simulink model "eVTOL_System"  (R2024b)
settings: Solver=FixedStepAuto  StartTime=0.0  StopTime=inf  RelTol=1e-3
undefined symbols (not defined in the file): airspeed, Battery, BCE12, BCE_Set_init, BMS_Controller_State, C, Cell10_P, Cell11_P, Cell12_P, Cell13_P, Cell14_P, Cell15_P, Cell16_P, Cell17_P, Cell18_P, Cell19_P, Cell1_N, Cell1_P, Cell20_P, Cell21_P, Cell22_P, Cell23_P, Cell24_P, Cell2_P, Cell3_P, Cell4_P, Cell5_P, Cell6_P, Cell7_P, Cell8_P, Cell9_P, Charging_State, CityMission, control, controlParams, ControlSampleTime, CriticalTiltAngle, currentFactor, CV_Gain, ddx, ddy, ddz, Device_01, Device_02, DiscIntNeverNeededParam, dx, dy, dz, Earth, env, F, F28379D_ADC_MaxCount, F28379D_ADC_Vmax, FixedWingMission, flightState, Foc_Ki_IxTcpu, Foc_Ki_S, Foc_Kp_I, Foc_Kp_S, fractalcoef ... (+68)
libraries: fl_lib x1115, nesl_utility x617, slrealtimeethercatlib x217, simulink x130, canmsglib x101, speedgoatlib_IO611_obsolete x91, slpidlib x49, mcbcontrolslib x44, slrealtimeutilitieslib x35, speedgoatlib_hdlCoder_IO3xx x31, dspstat3 x24, mcbpositiondecoderlib x12
(part 1 of 31)
settings Model: DataDictionary=VTOLDynamicsData.sldd  Creator=The MathWorks, Inc.  LastModifiedBy=jatin.anand
settings SolverCC: ConcurrentTasks=on  PositivePriorityOrder=on  AutoInsertRateTranBlk=on
settings OptimizationCC: BlockReduction=off  OptimizeBlockIOStorage=off  EnhancedBackFolding=on  PassReuseOutputArgsThreshold=0  OptimizeBlockOrder=speed  DifferentSizesBufferReuse=on
settings DebuggingCC: TasksWithSamePriorityMsg=none  ParameterTunabilityLossMsg=error
settings HardwareCC: ProdBitPerLong=64  ProdLongLongMode=on  ProdHWDeviceType=Intel->x86-64 (Linux 64)
settings RTWCC: Description=Speedgoat Real-Time Target Machine  SystemTargetFile=speedgoat.tlc  TemplateMakefile=slrealtime_default_tmf  Toolchain=Simulink Real-Time Toolchain  BuildConfiguration=Faster Runs  CodeExecutionProfiling=on  TargetLang=C++  GPUComputeCapability=3.5
settings CodeAppCC: ForceParamTrailComments=on  OperatorAnnotations=on
settings SimulinkRealTimeTargetCC: InstructionSetFMA=off  LogToMDFFile=off

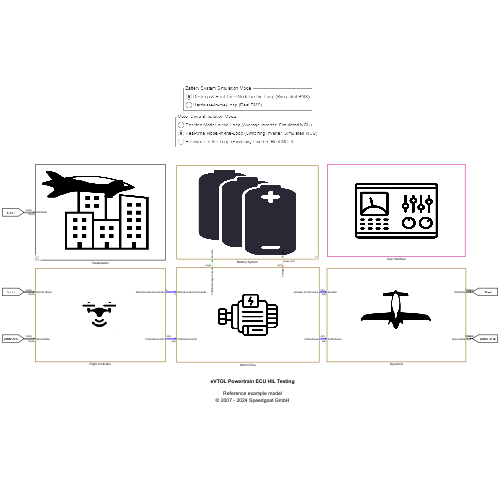
[thumbnail: Simulink's stored preview of the top-level diagram]
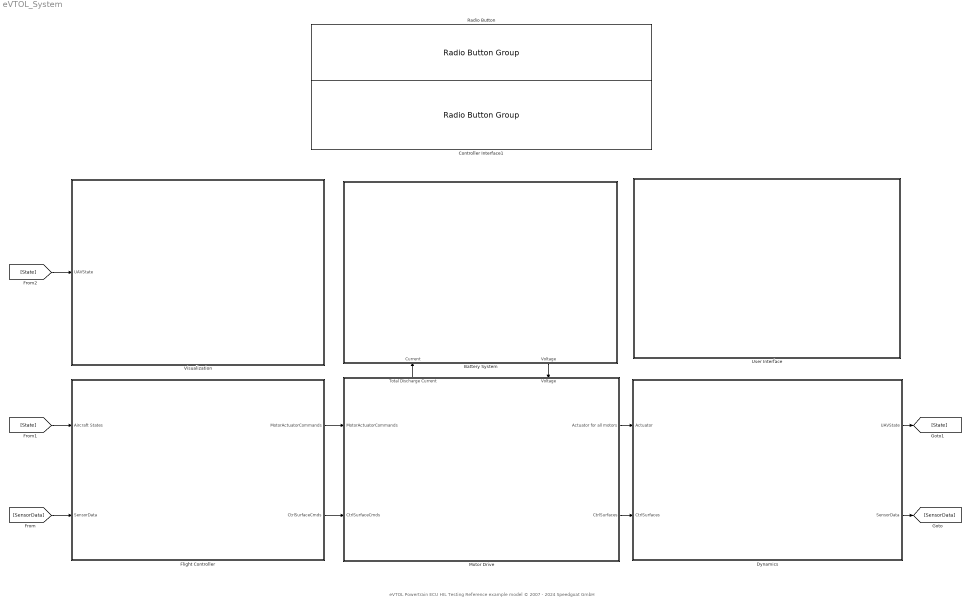
== system eVTOL_System ==
  note: eVTOL Powertrain ECU HIL Testing
      |
      | Reference example model
      | © 2007 - 2024 Speedgoat GmbH
  Battery System : Subsystem
      settings: PortSchema="{\"entries\":[{\"content\":{\"sides\":[{\"content\":{},\"type\":\"ConnectorPlacement.EquallySpacedRectSide\",\"uuid\":\"31833601-2311-4886-a109-2c0986e73e51\"},{\"content\":{\"side\":\"RIGHT\"},\"type\":\"ConnectorPlacement.EquallySpacedRectSide\",\"uuid\":\"85d08f94-66a0-4dc1-8c2a-87d8bd35677a\"},{\"content\":{\"side\":\"TOP\"},\"type\":\"ConnectorPlacement.EquallySpacedRectSide\",\"uuid\":\"8127f2a5-c494-4abc-920f-c6b2b4ea5251\"},{\"content\":{\"connectorIds\":[\"In1\",\"Out1\"],\"side\":\"BOTTOM\"},\"type\":\"ConnectorPlacement.EquallySpacedRectSide\",\"uuid\":\"983fb099-1c21-4d2b-9dd6-d2e6655b3784\"}]},\"type\":\"ConnectorPlacement.EquallySpacedConnector\",\"uuid\":\"c8b985e5-7cab-42e7-873f-ff2e7ab90a73\"}],\"packageUris\":[\"http://schema.mathworks.com/mf0/Connector/R2020b\"],\"version\":\"1.0\"}"
      mask Display: image('Battery.png');
  Controller Interface1 : RadioButtonGroup  LabelPosition=Hide  SelectedLabel=Real-time Model-in-the-Loop (Switching Inverter, Simulated MCU)  ButtonGroupName=Motor Drive Simulation Mode
      settings: Values={{'Desktop Model-in-the-Loop (Average Inverter, Simulated MCU)', 'Real-time Model-in-the-Loop (Switching Inverter, Simulated MCU)', 'Hardware-in-the-Loop (Switching Inverter, Real MCU)'}, [1 2 3]}
  Dynamics : Subsystem
      mask Display: image('fLIGHT_dYNAMICS.png', [0,0,0,0,80,80]);
  Flight Controller : Subsystem
      mask Display: image('Flight.png', [0,0,0,0,40,40]);
  Motor Drive : Subsystem
      settings: PortSchema="{\"entries\":[{\"content\":{\"sides\":[{\"content\":{\"connectorIds\":[\"In1\",\"In2\"]},\"type\":\"ConnectorPlacement.EquallySpacedRectSide\",\"uuid\":\"8efb4856-e5e8-4119-b327-f21a1b3c8e4f\"},{\"content\":{\"connectorIds\":[\"Out1\",\"Out2\"],\"side\":\"RIGHT\"},\"type\":\"ConnectorPlacement.EquallySpacedRectSide\",\"uuid\":\"1db0dfc6-79ae-47c2-8aa8-e6c666fa7b0e\"},{\"content\":{\"connectorIds\":[\"Out3\",\"In3\"],\"side\":\"TOP\"},\"type\":\"ConnectorPlacement.EquallySpacedRectSide\",\"uuid\":\"2682ef6f-b09c-4157-ad22-73f596ffc247\"}]},\"type\":\"ConnectorPlacement.EquallySpacedConnector\",\"uuid\":\"885b870f-d4fa-4030-b106-4e1ba5f331f5\"}],\"packageUris\":[\"http://schema.mathworks.com/mf0/Connector/R2020b\"],\"version\":\"1.0\"}"
      mask Display: image('PmsmMask.png');
  Radio Button : RadioButtonGroup  LabelPosition=Hide  SelectedLabel=Desktop & Real-Time Model-in-the-Loop (Simulated BMS)  ButtonGroupName=Battery System Simulation Mode
      settings: Values={{'Desktop & Real-Time Model-in-the-Loop (Simulated BMS)', 'Hardware-in-the-Loop (Real BMS)'}, [0 1]}
  User Interface : Subsystem
      mask Display: image('UIMask.png');
  Visualization : Subsystem  Variant=on  VariantControl=Visualization
      mask Display: image('3DVisualization.png');
  wires:
  Dynamics/2(SensorData) -> [SensorData]
  [SensorData] -> Flight Controller/2(SensorData)
  [State] -> Flight Controller/1(Aircraft States)
  [State] -> Visualization/1(UAVState)
  Flight Controller/1(MotorActuatorCommands) -> Motor Drive/1(MotorActuatorCommands)
  Flight Controller/2(CtrlSurfaceCmds) -> Motor Drive/2(CtrlSurfaceCmds)
  Motor Drive/1(Actuator for all motors) -> Dynamics/1(Actuator)
  Motor Drive/2(CtrlSurfaces) -> Dynamics/2(CtrlSurfaces)
  Battery System/1(Voltage) -> Motor Drive/3(Voltage)
  Dynamics/1(UAVState) -> [State]
  Motor Drive/3(Total Discharge Current) -> Battery System/1(Current)

== system eVTOL_System/Battery System ==
  note: Battery Management System HIL
      |
      | Reference example model
      | © 2007 - 2024 Speedgoat GmbH
  Current : Inport
  BMS : Subsystem  Variant=on  VariantControl=Choice
      mask Display: image('BMS.png'); % Use "Edit Image" on toolstrip to change.
  Battery : Subsystem
      mask Display: image('battery.png'); % Use "Edit Image" on toolstrip to change.
  Instrumentation : Subsystem
      mask Display: image('tunable.png'); % Use "Edit Image" on toolstrip to change.
  Voltage : Outport
  tag scope: Controller_Info=global, Controller_Output=global, Sensor_Values=global
  wires:
  [Voltage] -> Voltage/1
  [State_Request] -> BMS/1(State_Request)
  [Current_Request] -> Battery/1(Current_Request)
  BMS/1(Controller_Info) -> [Controller_Info]  "Controller_Info"
  Battery/1(Sensor_Values) -> [Sensor_Values]
  BMS/2(Controller_Output) -> [Controller_Output]  "Controller_Output"
  Current/1 -> Instrumentation/1(Current)
  [Sensor_Values] -> BMS/2(Sensor_Values)
  connections:
  Battery/RConn1 -- BMS/LConn1
  Battery/RConn2 -- BMS/LConn2
  Battery/RConn3 -- BMS/LConn3

== system eVTOL_System/Dynamics ==
  note: Forces and Moments - VTOL UAV plant model and weather model
      | 6DOF (Euler Angles Conversion) - Converts forces and moments from body to inertial frame
      | Ground Truth Bus - converts UAV States into bus
  Actuator : Inport
  CtrlSurfaces : Inport  Port=2
  6DOF (Euler Angles)1 : shared6dof/6DOF (Euler Angles)  units=Metric (MKS)  mtype=Fixed  rep=Euler Angles  xme_0=[xGround, yGround, zGround]  Vm_0=[vIni 0 0]  eul_0=[iniRoll initPitch iniYaw]  pm_0=[0 0 0]  mass_0=6.031  mass_e=0.5  mass_f=2.0  inertia=[uavParam.geom.Ixx 0 0; 0 uavParam.geom.Iyy 0; 0 0 uavParam.geom.Izz]  inertia_e=eye(3)  inertia_f=2*eye(3)  k_quat=1.0  vre_flag=on  abi_flag=on  aMode=0  xme_statename=''  Vm_statename=''  eul_statename=''  quat_statename=''  pm_statename=''  mass_statename=''
  Bus Selector : BusSelector  OutputSignals=RotorParameters.w1,RotorParameters.w2,RotorParameters.w3,RotorParameters.w4
  Force and Moments : Subsystem
  Ground Truth Bus : Subsystem
  Scope : Scope  NumInputPorts=4
  Terminator : Terminator
  Variant Subsystem : Subsystem  Variant=on  VariantControl=Choice
  UAVState : Outport
  SensorData : Outport  Port=2
  wires:
  Force and Moments/1(F) -> 6DOF (Euler Angles)1/1
  Force and Moments/2(M) -> 6DOF (Euler Angles)1/2
  Actuator/1 -> Force and Moments/1(Actuator)
  CtrlSurfaces/1 -> Force and Moments/2(CtrlSurfaces)
  6DOF (Euler Angles)1/1 -> Ground Truth Bus/1(Ve)  "Ve"
  6DOF (Euler Angles)1/2 -> Ground Truth Bus/2(Xe)  "Xe"
  6DOF (Euler Angles)1/3 -> Ground Truth Bus/3(Euler)  "Euler"
  6DOF (Euler Angles)1/4 -> Ground Truth Bus/4(DCMbe)  "DCMbe"
  6DOF (Euler Angles)1/5 -> Ground Truth Bus/5(Vb)  "Vb"
  6DOF (Euler Angles)1/6 -> Ground Truth Bus/6(pqr)  "pqr"
  6DOF (Euler Angles)1/7 -> Terminator/1
  6DOF (Euler Angles)1/8 -> Ground Truth Bus/7(Abb)  "Abb"
  Force and Moments/3(RotorParams) -> Ground Truth Bus/9(RotorParams)  "RotorParams"
  Force and Moments/4(AirData) -> Ground Truth Bus/10(AirData)
  Variant Subsystem/1(SensorData) -> SensorData/1
  6DOF (Euler Angles)1/9 -> Ground Truth Bus/8(Abe)
  Ground Truth Bus/1(Ground Truth) -> Bus Selector/1, UAVState/1, Force and Moments/3(States), Variant Subsystem/1(UAVStates)  "Ground Truth"
  Bus Selector/1 -> Scope/1  "<w1>"
  Bus Selector/2 -> Scope/2  "<w2>"
  Bus Selector/3 -> Scope/3  "<w3>"
  Bus Selector/4 -> Scope/4  "<w4>"

== system eVTOL_System/Flight Controller ==
  Aircraft States : Inport
  SensorData : Inport  Port=2
  Autopilot : Subsystem
  Estimator : Subsystem  Variant=on
  Ground Control Station : Subsystem
  Guidance Test Bench : Subsystem
  MotorActuatorCommands : Outport
  CtrlSurfaceCmds : Outport  Port=2
  wires:
  Guidance Test Bench/3(AACSP) -> Autopilot/3(AAC)
  Estimator/1(EstimatedStates) -> Autopilot/6(EstimatedStates), Ground Control Station/1(UAVState)
  Ground Control Station/1(Global Mission) -> Guidance Test Bench/2(Global Mission)
  Guidance Test Bench/5(FlightMode) -> Autopilot/5(FlightMode)
  Guidance Test Bench/1(HoverSP) -> Autopilot/1(HoverCommands)
  Guidance Test Bench/2(FixedWingSP) -> Autopilot/2(FixedWingSP)
  SensorData/1 -> Estimator/1(SensorData)
  Guidance Test Bench/4(ctrlMode) -> Autopilot/4(CtrlMode)
  Autopilot/1(MotorActuatorCommands) -> MotorActuatorCommands/1
  Autopilot/2(CtrlSurfaceCmds) -> CtrlSurfaceCmds/1
  Aircraft States/1 -> Guidance Test Bench/1(Aircraft States)

== system eVTOL_System/Motor Drive ==
  MotorActuatorCommands : Inport
  CtrlSurfaceCmds : Inport  Port=2
  Voltage : Inport  Port=3
  Actuator To PWM for all motors : Subsystem
  Actuator To RPM for 1 motor : Subsystem
  Actuator To RPM for 1 motor1 : Subsystem
  Actuator To RPM for 1 motor2 : Subsystem
  Actuator To RPM for 1 motor3 : Subsystem
  Add : Sum  Inputs=++++
  Closed_Loop_FOC{,1..3} (4 alike) : Constant  OutDataTypeStr=boolean  SampleTime=Ts_UI
  Controller : Subsystem  Variant=on  VariantControl=Choice
      settings: PortSchema="{\"entries\":[{\"content\":{\"sides\":[{\"content\":{\"connectorIds\":[\"In1\",\"In2\",\"In3\",\"In4\",\"In5\",\"In6\"]},\"type\":\"ConnectorPlacement.EquallySpacedRectSide\",\"uuid\":\"39f08c92-b87f-4f95-877f-fef0e466fbdb\"},{\"content\":{\"connectorIds\":[\"Out1\"],\"side\":\"RIGHT\"},\"type\":\"ConnectorPlacement.EquallySpacedRectSide\",\"uuid\":\"6fadd6f2-7db3-41c1-89a7-be1692c18c49\"},{\"content\":{\"connectorIds\":[\"Out2\"],\"side\":\"TOP\"},\"type\":\"ConnectorPlacement.EquallySpacedRectSide\",\"uuid\":\"aea4ee68-7094-4bdc-b416-2d8969306971\"}]},\"type\":\"ConnectorPlacement.EquallySpacedConnector\",\"uuid\":\"e129f01f-1291-4735-8ea4-164650c1b4f8\"}],\"packageUris\":[\"http://schema.mathworks.com/mf0/Connector/R2020b\"],\"version\":\"1.0\"}"
      mask Display: image('MCUMask.png');
  Controller Parameters : Subsystem
  Controller Parameters1 : Subsystem
  Controller Parameters2 : Subsystem
  Controller Parameters3 : Subsystem
  Controller1 : Subsystem  Variant=on  VariantControl=Choice
      settings: PortSchema="{\"entries\":[{\"content\":{\"sides\":[{\"content\":{\"connectorIds\":[\"In1\",\"In2\",\"In3\",\"In4\",\"In5\",\"In6\"]},\"type\":\"ConnectorPlacement.EquallySpacedRectSide\",\"uuid\":\"39f08c92-b87f-4f95-877f-fef0e466fbdb\"},{\"content\":{\"connectorIds\":[\"Out1\"],\"side\":\"RIGHT\"},\"type\":\"ConnectorPlacement.EquallySpacedRectSide\",\"uuid\":\"6fadd6f2-7db3-41c1-89a7-be1692c18c49\"},{\"content\":{\"connectorIds\":[\"Out2\"],\"side\":\"TOP\"},\"type\":\"ConnectorPlacement.EquallySpacedRectSide\",\"uuid\":\"aea4ee68-7094-4bdc-b416-2d8969306971\"}]},\"type\":\"ConnectorPlacement.EquallySpacedConnector\",\"uuid\":\"e129f01f-1291-4735-8ea4-164650c1b4f8\"}],\"packageUris\":[\"http://schema.mathworks.com/mf0/Connector/R2020b\"],\"version\":\"1.0\"}"
      mask Display: image('MCUMask.png');
  Controller2 : Subsystem  Variant=on  VariantControl=Choice
      settings: PortSchema="{\"entries\":[{\"content\":{\"sides\":[{\"content\":{\"connectorIds\":[\"In1\",\"In2\",\"In3\",\"In4\",\"In5\",\"In6\"]},\"type\":\"ConnectorPlacement.EquallySpacedRectSide\",\"uuid\":\"39f08c92-b87f-4f95-877f-fef0e466fbdb\"},{\"content\":{\"connectorIds\":[\"Out1\"],\"side\":\"RIGHT\"},\"type\":\"ConnectorPlacement.EquallySpacedRectSide\",\"uuid\":\"6fadd6f2-7db3-41c1-89a7-be1692c18c49\"},{\"content\":{\"connectorIds\":[\"Out2\"],\"side\":\"TOP\"},\"type\":\"ConnectorPlacement.EquallySpacedRectSide\",\"uuid\":\"aea4ee68-7094-4bdc-b416-2d8969306971\"}]},\"type\":\"ConnectorPlacement.EquallySpacedConnector\",\"uuid\":\"e129f01f-1291-4735-8ea4-164650c1b4f8\"}],\"packageUris\":[\"http://schema.mathworks.com/mf0/Connector/R2020b\"],\"version\":\"1.0\"}"
      mask Display: image('MCUMask.png');
  Controller3 : Subsystem  Variant=on  VariantControl=Choice
      settings: PortSchema="{\"entries\":[{\"content\":{\"sides\":[{\"content\":{\"connectorIds\":[\"In1\",\"In2\",\"In3\",\"In4\",\"In5\",\"In6\"]},\"type\":\"ConnectorPlacement.EquallySpacedRectSide\",\"uuid\":\"39f08c92-b87f-4f95-877f-fef0e466fbdb\"},{\"content\":{\"connectorIds\":[\"Out1\"],\"side\":\"RIGHT\"},\"type\":\"ConnectorPlacement.EquallySpacedRectSide\",\"uuid\":\"6fadd6f2-7db3-41c1-89a7-be1692c18c49\"},{\"content\":{\"connectorIds\":[\"Out2\"],\"side\":\"TOP\"},\"type\":\"ConnectorPlacement.EquallySpacedRectSide\",\"uuid\":\"aea4ee68-7094-4bdc-b416-2d8969306971\"}]},\"type\":\"ConnectorPlacement.EquallySpacedConnector\",\"uuid\":\"e129f01f-1291-4735-8ea4-164650c1b4f8\"}],\"packageUris\":[\"http://schema.mathworks.com/mf0/Connector/R2020b\"],\"version\":\"1.0\"}"
      mask Display: image('MCUMask.png');
  Controller_fbk_signals : Subsystem
  Controller_fbk_signals1 : Subsystem
  Controller_fbk_signals2 : Subsystem
  Controller_fbk_signals3 : Subsystem
  Data Type Conversion{,1..3} (4 alike) : DataTypeConversion  OutDataTypeStr=single  SaturateOnIntegerOverflow=off  RndMeth=Floor
  Delay{,1..3} (4 alike) : Delay
  EnablePWM{,1..3} (4 alike) : Constant  OutDataTypeStr=boolean  SampleTime=Ts_UI
  Fault Trigering : Subsystem
  Fault Trigering1 : Subsystem
  Fault Trigering2 : Subsystem
  Fault Trigering3 : Subsystem
  Load{,1..3} (4 alike) : Constant  Value=0  OutDataTypeStr=single
  Motor Model Feedback : Subsystem
  Motor Model Feedback1 : Subsystem
  Motor Model Feedback2 : Subsystem
  Motor Model Feedback3 : Subsystem
  Mux{,1..3} (4 alike) : Mux  Inputs=2
  SimulationVariant : Constant  Value=2
  Terminator{,1..4} (5 alike) : Terminator
  Three-Phase PMSM Drive : Subsystem  Variant=on  VariantControl=Choice
      settings: PortSchema="{\"entries\":[{\"content\":{\"sides\":[{\"content\":{\"connectorIds\":[\"In1\",\"In2\",\"In3\"]},\"type\":\"ConnectorPlacement.EquallySpacedRectSide\",\"uuid\":\"be3bef0c-fa0d-49a9-8d81-4a9438f9f09e\"},{\"content\":{\"connectorIds\":[\"Out1\",\"Out2\",\"Out3\",\"Out4\",\"Out5\",\"Out6\"],\"side\":\"RIGHT\"},\"type\":\"ConnectorPlacement.EquallySpacedRectSide\",\"uuid\":\"a97c4291-bd47-47ae-a87a-e148291abc4a\"},{\"content\":{\"connectorIds\":[\"In4\"],\"side\":\"TOP\"},\"type\":\"ConnectorPlacement.EquallySpacedRectSide\",\"uuid\":\"93bcf0c4-5b44-4ac3-b6c3-6b4577237bd1\"}]},\"type\":\"ConnectorPlacement.EquallySpacedConnector\",\"uuid\":\"9c4ab161-5f4a-4191-8213-47b9045836c1\"}],\"packageUris\":[\"http://schema.mathworks.com/mf0/Connector/R2020b\"],\"version\":\"1.0\"}"
      mask Display: image('pmsmMask.png'); % Use "Edit Image" on toolstrip to change.
  Three-Phase PMSM Drive1 : Subsystem  Variant=on  VariantControl=Choice
      settings: PortSchema="{\"entries\":[{\"content\":{\"sides\":[{\"content\":{\"connectorIds\":[\"In1\",\"In2\",\"In3\"]},\"type\":\"ConnectorPlacement.EquallySpacedRectSide\",\"uuid\":\"be3bef0c-fa0d-49a9-8d81-4a9438f9f09e\"},{\"content\":{\"connectorIds\":[\"Out1\",\"Out2\",\"Out3\",\"Out4\",\"Out5\",\"Out6\"],\"side\":\"RIGHT\"},\"type\":\"ConnectorPlacement.EquallySpacedRectSide\",\"uuid\":\"a97c4291-bd47-47ae-a87a-e148291abc4a\"},{\"content\":{\"connectorIds\":[\"In4\"],\"side\":\"TOP\"},\"type\":\"ConnectorPlacement.EquallySpacedRectSide\",\"uuid\":\"93bcf0c4-5b44-4ac3-b6c3-6b4577237bd1\"}]},\"type\":\"ConnectorPlacement.EquallySpacedConnector\",\"uuid\":\"9c4ab161-5f4a-4191-8213-47b9045836c1\"}],\"packageUris\":[\"http://schema.mathworks.com/mf0/Connector/R2020b\"],\"version\":\"1.0\"}"
      mask Display: image('pmsmMask.png'); % Use "Edit Image" on toolstrip to change.
  Three-Phase PMSM Drive2 : Subsystem  Variant=on  VariantControl=Choice
      settings: PortSchema="{\"entries\":[{\"content\":{\"sides\":[{\"content\":{\"connectorIds\":[\"In1\",\"In2\",\"In3\"]},\"type\":\"ConnectorPlacement.EquallySpacedRectSide\",\"uuid\":\"be3bef0c-fa0d-49a9-8d81-4a9438f9f09e\"},{\"content\":{\"connectorIds\":[\"Out1\",\"Out2\",\"Out3\",\"Out4\",\"Out5\",\"Out6\"],\"side\":\"RIGHT\"},\"type\":\"ConnectorPlacement.EquallySpacedRectSide\",\"uuid\":\"a97c4291-bd47-47ae-a87a-e148291abc4a\"},{\"content\":{\"connectorIds\":[\"In4\"],\"side\":\"TOP\"},\"type\":\"ConnectorPlacement.EquallySpacedRectSide\",\"uuid\":\"93bcf0c4-5b44-4ac3-b6c3-6b4577237bd1\"}]},\"type\":\"ConnectorPlacement.EquallySpacedConnector\",\"uuid\":\"9c4ab161-5f4a-4191-8213-47b9045836c1\"}],\"packageUris\":[\"http://schema.mathworks.com/mf0/Connector/R2020b\"],\"version\":\"1.0\"}"
      mask Display: image('pmsmMask.png'); % Use "Edit Image" on toolstrip to change.
  Three-Phase PMSM Drive3 : Subsystem  Variant=on  VariantControl=Choice
      settings: PortSchema="{\"entries\":[{\"content\":{\"sides\":[{\"content\":{\"connectorIds\":[\"In1\",\"In2\",\"In3\"]},\"type\":\"ConnectorPlacement.EquallySpacedRectSide\",\"uuid\":\"be3bef0c-fa0d-49a9-8d81-4a9438f9f09e\"},{\"content\":{\"connectorIds\":[\"Out1\",\"Out2\",\"Out3\",\"Out4\",\"Out5\",\"Out6\"],\"side\":\"RIGHT\"},\"type\":\"ConnectorPlacement.EquallySpacedRectSide\",\"uuid\":\"a97c4291-bd47-47ae-a87a-e148291abc4a\"},{\"content\":{\"connectorIds\":[\"In4\"],\"side\":\"TOP\"},\"type\":\"ConnectorPlacement.EquallySpacedRectSide\",\"uuid\":\"93bcf0c4-5b44-4ac3-b6c3-6b4577237bd1\"}]},\"type\":\"ConnectorPlacement.EquallySpacedConnector\",\"uuid\":\"9c4ab161-5f4a-4191-8213-47b9045836c1\"}],\"packageUris\":[\"http://schema.mathworks.com/mf0/Connector/R2020b\"],\"version\":\"1.0\"}"
      mask Display: image('pmsmMask.png'); % Use "Edit Image" on toolstrip to change.
  Actuator for all motors : Outport
  CtrlSurfaces : Outport  Port=2
  Total Discharge Current : Outport  Port=3
  wires:
  CtrlSurfaceCmds/1 -> CtrlSurfaces/1
  SimulationVariant/1 -> Terminator2/1
  Controller/1(Controller_fbk) -> Controller_fbk_signals/1(Controller_fbk)
  [Iab1] -> Controller/1(Iab)
  Three-Phase PMSM Drive/4(Motor_Spd) -> Motor Model Feedback/4(Motor_SPD_rads)
  Three-Phase PMSM Drive/3(Ic) -> Motor Model Feedback/3(Ic)
  [QAE_Pos_C1] -> Controller/2(QAE_MIL_fbk)
  Three-Phase PMSM Drive/2(Ib) -> Mux/2, Motor Model Feedback/2(Ib)
  Controller Parameters/1(Controller Parameters) -> Controller/6(Controller_Parameters)
  Three-Phase PMSM Drive/1(Ia) -> Mux/1, Motor Model Feedback/1(Ia)
  EnablePWM/1 -> Controller/3(EnablePWM)
  Three-Phase PMSM Drive/5(Motor_Angle) -> Terminator/1
  Load/1 -> Three-Phase PMSM Drive/3(LdTrq/Spd)
  Mux/1 -> [Iab1]
  Closed_Loop_FOC/1 -> Controller/4(Closed_Loop_FOC)
  Fault Trigering/1(Faults) -> Three-Phase PMSM Drive/2(Fault)
  Three-Phase PMSM Drive/6(QAE_Pos_C) -> [QAE_Pos_C1]
  Controller/2(Simu_config) -> Three-Phase PMSM Drive/4(Simu_config)
  Actuator To PWM for all motors/1(To PWM) -> Actuator for all motors/1
  Data Type Conversion/1 -> Controller/5(Speed_CMD_RPM)
  Three-Phase PMSM Drive1/5(Motor_Angle) -> Terminator1/1
  Load1/1 -> Three-Phase PMSM Drive1/3(LdTrq/Spd)
  Three-Phase PMSM Drive1/4(Motor_Spd) -> Motor Model Feedback1/4(Motor_SPD_rads)
  [Iab2] -> Controller1/1(Iab)
  Three-Phase PMSM Drive1/3(Ic) -> Motor Model Feedback1/3(Ic)
  Mux1/1 -> [Iab2]
  Three-Phase PMSM Drive1/2(Ib) -> Mux1/2, Motor Model Feedback1/2(Ib)
  Data Type Conversion1/1 -> Controller1/5(Speed_CMD_RPM)
  Controller Parameters1/1(Controller Parameters) -> Controller1/6(Controller_Parameters)
  Three-Phase PMSM Drive1/6(QAE_Pos_C) -> [QAE_Pos_C2]
  [QAE_Pos_C2] -> Controller1/2(QAE_MIL_fbk)
  Controller1/2(Simu_config) -> Three-Phase PMSM Drive1/4(Simu_config)
  Fault Trigering1/1(Faults) -> Three-Phase PMSM Drive1/2(Fault)
  EnablePWM1/1 -> Controller1/3(EnablePWM)
  Closed_Loop_FOC1/1 -> Controller1/4(Closed_Loop_FOC)
  Controller1/1(Controller_fbk) -> Controller_fbk_signals1/1(Controller_fbk)
  Three-Phase PMSM Drive1/1(Ia) -> Mux1/1, Motor Model Feedback1/1(Ia)
  Actuator To RPM for 1 motor1/1(RPM) -> Data Type Conversion1/1
  Controller2/1(Controller_fbk) -> Controller_fbk_signals2/1(Controller_fbk)
  Closed_Loop_FOC2/1 -> Controller2/4(Closed_Loop_FOC)
  Fault Trigering2/1(Faults) -> Three-Phase PMSM Drive2/2(Fault)
  Three-Phase PMSM Drive2/6(QAE_Pos_C) -> [QAE_Pos_C3]
  Actuator To RPM for 1 motor2/1(RPM) -> Data Type Conversion2/1
  Controller Parameters2/1(Controller Parameters) -> Controller2/6(Controller_Parameters)
  Data Type Conversion2/1 -> Controller2/5(Speed_CMD_RPM)
  Three-Phase PMSM Drive2/1(Ia) -> Mux2/1, Motor Model Feedback2/1(Ia)
  Controller2/2(Simu_config) -> Three-Phase PMSM Drive2/4(Simu_config)
  [QAE_Pos_C3] -> Controller2/2(QAE_MIL_fbk)
  Three-Phase PMSM Drive2/2(Ib) -> Mux2/2, Motor Model Feedback2/2(Ib)
  [Iab3] -> Controller2/1(Iab)
  Three-Phase PMSM Drive2/3(Ic) -> Motor Model Feedback2/3(Ic)
  Load2/1 -> Three-Phase PMSM Drive2/3(LdTrq/Spd)
  Three-Phase PMSM Drive2/4(Motor_Spd) -> Motor Model Feedback2/4(Motor_SPD_rads)
  Mux2/1 -> [Iab3]
  EnablePWM2/1 -> Controller2/3(EnablePWM)
  Three-Phase PMSM Drive2/5(Motor_Angle) -> Terminator3/1
  Controller3/1(Controller_fbk) -> Controller_fbk_signals3/1(Controller_fbk)
  Closed_Loop_FOC3/1 -> Controller3/4(Closed_Loop_FOC)
  Fault Trigering3/1(Faults) -> Three-Phase PMSM Drive3/2(Fault)
  Three-Phase PMSM Drive3/6(QAE_Pos_C) -> [QAE_Pos_C4]
  Actuator To RPM for 1 motor3/1(RPM) -> Data Type Conversion3/1
  Controller Parameters3/1(Controller Parameters) -> Controller3/6(Controller_Parameters)
  Data Type Conversion3/1 -> Controller3/5(Speed_CMD_RPM)
  Three-Phase PMSM Drive3/1(Ia) -> Mux3/1, Motor Model Feedback3/1(Ia)
  Controller3/2(Simu_config) -> Three-Phase PMSM Drive3/4(Simu_config)
  [QAE_Pos_C4] -> Controller3/2(QAE_MIL_fbk)
  Three-Phase PMSM Drive3/2(Ib) -> Mux3/2, Motor Model Feedback3/2(Ib)
  [Iab4] -> Controller3/1(Iab)
  Three-Phase PMSM Drive3/3(Ic) -> Motor Model Feedback3/3(Ic)
  Load3/1 -> Three-Phase PMSM Drive3/3(LdTrq/Spd)
  Three-Phase PMSM Drive3/4(Motor_Spd) -> Motor Model Feedback3/4(Motor_SPD_rads)
  Mux3/1 -> [Iab4]
  EnablePWM3/1 -> Controller3/3(EnablePWM)
  Three-Phase PMSM Drive3/5(Motor_Angle) -> Terminator4/1
  MotorActuatorCommands/1 -> Actuator To RPM for 1 motor1/1(Motor Commands), Actuator To RPM for 1 motor2/1(Motor Commands), Actuator To RPM for 1 motor3/1(Motor Commands), Actuator To PWM for all motors/1(Motor Commands), Actuator To RPM for 1 motor/1(Motor Commands)
  [Idc4] -> Delay3/1
  [Idc3] -> Delay2/1
  [Idc2] -> Delay1/1
  [Idc1] -> Delay/1
  Add/1 -> Total Discharge Current/1
  Delay/1 -> Add/1
  Delay1/1 -> Add/2
  Delay2/1 -> Add/3
  Delay3/1 -> Add/4
  Actuator To RPM for 1 motor/1(RPM) -> Data Type Conversion/1
  Voltage/1 -> Three-Phase PMSM Drive3/1(V_dc), Three-Phase PMSM Drive2/1(V_dc), Three-Phase PMSM Drive1/1(V_dc), Three-Phase PMSM Drive/1(V_dc)

== system eVTOL_System/User Interface ==
  " System User Interface" : Subsystem
      mask Display: image('UIMask.png');
  BMS User Interface : Subsystem
      mask Display: image('UIMask.png');
  Motor Drive User Interface : Subsystem
      mask Display: image('UIMask.png');

== system eVTOL_System/Visualization ==
  UAVState : Inport
  No Visualization : Subsystem  VariantControl=Visualization==0
  Photorealistic : Subsystem  Variant=on  VariantControl=Visualization==2
  Visualization : Subsystem  Variant=on  VariantControl=Visualization==1

== system eVTOL_System/Battery System/BMS ==
  State_Request : Inport
  Sensor_Values : Inport  Port=2
  HIL : Subsystem  VariantControl=strcmp(get_param(['eVTOL_System/Battery System/Instrumentation/Simulation_Profile_Value'], 'Value'),'1')
  MIL : Subsystem  VariantControl=strcmp(get_param(['eVTOL_System/Battery System/Instrumentation/Simulation_Profile_Value'], 'Value'),'0')
  Cells : PMIOPort  Side=Left
  Cells1 : PMIOPort  Port=2  Side=Left
  Cells2 : PMIOPort  Port=3  Side=Left
  Controller_Info : Outport
  Controller_Output : Outport  Port=2

== system eVTOL_System/Battery System/Battery ==
  Current_Request : Inport
  Battery Pack : Subsystem
  Bus Creator1 : BusCreator  Inputs=6
  Data Type Conversion{,1..3,6..7} (6 alike) : DataTypeConversion  OutDataTypeStr=single  SaturateOnIntegerOverflow=off  RndMeth=Floor
  Electrical Interface : Subsystem
      settings: PortSchema="{\"entries\":[{\"content\":{\"sides\":[{\"content\":{\"connectorIds\":[\"LConn1\",\"LConn2\"]},\"type\":\"ConnectorPlacement.EquallySpacedRectSide\",\"uuid\":\"060ff703-e9b3-40ce-a787-2ee59c0c5ac0\"},{\"content\":{\"connectorIds\":[\"Out1\",\"Out2\"],\"side\":\"RIGHT\"},\"type\":\"ConnectorPlacement.EquallySpacedRectSide\",\"uuid\":\"8c9bb67a-bc70-410b-a295-07dda5ac66bb\"},{\"content\":{\"side\":\"TOP\"},\"type\":\"ConnectorPlacement.EquallySpacedRectSide\",\"uuid\":\"38660739-cfc2-45c9-bc16-eb56669afec1\"},{\"content\":{\"connectorIds\":[\"In1\"],\"side\":\"BOTTOM\"},\"type\":\"ConnectorPlacement.EquallySpacedRectSide\",\"uuid\":\"71db0731-26a1-4041-8f3c-8f442f4d5aa6\"}]},\"type\":\"ConnectorPlacement.EquallySpacedConnector\",\"uuid\":\"4bfbaf33-58df-40e3-8b4c-5be4570a9e05\"}],\"packageUris\":[\"http://schema.mathworks.com/mf0/Connector/R2020b\"],\"version\":\"1.0\"}"
  HW Interface : Subsystem  Variant=on  VariantControl=Choice
  Override : Subsystem
  Rate Transition1 : RateTransition  OutPortSampleTime=ts_system
  Cells : PMIOPort  Side=Right
  Cells1 : PMIOPort  Port=2  Side=Right
  Cells2 : PMIOPort  Port=3  Side=Right
  Sensor_Values : Outport
  tag scope: Cells_SOCs=global
  wires:
  Current_Request/1 -> Rate Transition1/1
  Electrical Interface/1(Pack_Current) -> Data Type Conversion2/1
  Electrical Interface/2(Pack_Voltage) -> Data Type Conversion1/1
  Data Type Conversion/1 -> Bus Creator1/1  "Cell_Voltages"
  Data Type Conversion1/1 -> Bus Creator1/4  "Pack_Voltage"
  Data Type Conversion2/1 -> Bus Creator1/3  "Pack_Current"
  Data Type Conversion3/1 -> Bus Creator1/2  "Cell_Temperatures"
  [Ambient_Temperature_User] -> Battery Pack/1(Ambient_Temperature)
  Battery Pack/1(Cell_Voltages) -> Data Type Conversion/1
  Battery Pack/2(Cell_Temperatures) -> Data Type Conversion3/1
  Battery Pack/3(Cell_SOCs) -> [Cells_SOCs]  "Cell_SOCs"
  HW Interface/1(Sensor_Values_Real) -> Sensor_Values/1
  Rate Transition1/1 -> Electrical Interface/1(Current_Request)
  Bus Creator1/1 -> Override/1(Input)
  [Pack_Voltage_76Cells] -> Data Type Conversion6/1
  [Pack_Voltage_24Cells] -> Data Type Conversion7/1
  Data Type Conversion6/1 -> Bus Creator1/6  "Pack_Voltage2"
  Data Type Conversion7/1 -> Bus Creator1/5  "Pack_Voltage1"
  Override/1(Output) -> HW Interface/1(Sensor_Values_Sim)
  connections:
  Battery Pack/RConn1 -- Electrical Interface/LConn1
  Battery Pack/RConn2 -- Electrical Interface/LConn2
  Battery Pack/RConn3 -- HW Interface/LConn1
  HW Interface/RConn1 -- Cells/RConn1
  Battery Pack/RConn4 -- Cells1/RConn1
  Cells2/RConn1 -- Battery Pack/RConn5

== system eVTOL_System/Battery System/Instrumentation ==
  Current : Inport
  Ambient_Temperature : Constant  Value=25  SampleTime=-1
  Celsius_to_Kelvin : Subsystem
  Constant1 : Constant
  Current Control : Subsystem
  Instrumented Signals : Subsystem
  Mux : Mux  Inputs=3
  Simulation_Profile_Value : Constant  Value=0
  State_Request : simulink/Sources/Enumerated Constant  OutDataTypeStr=Enum: SRE  Value=SRE(0)  SampleTime=inf
  Terminator1 : Terminator
  Terminator4 : Terminator
  Test_Mode_Selector : Constant  Value=TestMode
  tag scope: Ambient_Temperature_User=global, Current_Request=global, State_Request=global
  wires:
  Celsius_to_Kelvin/1(K) -> [Ambient_Temperature_User]
  Ambient_Temperature/1 -> Celsius_to_Kelvin/1(C)
  Constant1/1 -> Current Control/2(Current_Request_User_Bypass)
  Current Control/1(Current_Request) -> [Current_Request]  "Pack_Current_Request"
  State_Request/1 -> [State_Request]
  [Controller_Output] -> Instrumented Signals/1(Controller_Output), Current Control/4(Controller_Output)
  [Controller_Info] -> Instrumented Signals/2(Controller_Info), Current Control/3(Controller_Info)
  [Sensor_Values] -> Instrumented Signals/3(Sensor_Values)
  [Cells_SOCs] -> Instrumented Signals/5(Cells_SOCs)
  Simulation_Profile_Value/1 -> Terminator4/1
  Test_Mode_Selector/1 -> Terminator1/1
  [Balancing_Currents1] -> Mux/2
  [Balancing_Currents] -> Mux/1
  [Balancing_Currents2] -> Mux/3
  Mux/1 -> Instrumented Signals/4(Balancing_Currents)
  Current/1 -> Current Control/1(Current_Request_User)

== system eVTOL_System/Dynamics/Force and Moments ==
  note: Weather Model - Wind model is disabled by default. To enable wind model, run Wind = 0 and configure the wind model in the Weather Model subsystem.
      |
      | Aerodynamic Forces - Computes aerodynamic forces of the UAV. To modify the aerodynamic derivatives of the UAV, modify the uavParam.aero struct with your own data, or use the Aerodynamic Forces and Moments block from Aerospace Blockset
      |
      | Propulsion - Models the propulsion system. Open this subsystem to configure the rotor direction, tilt angle, etc.
  Actuator : Inport
  CtrlSurfaces : Inport  Port=2
  States : Inport  Port=3
  Add : Sum  Inputs=++++
  Add1 : Sum
  AeroSwitch : Constant  Value=0
  Aerodynamic Drag : Subsystem
  Aerodynamic Forces : Subsystem
  Bus Selector : BusSelector  OutputSignals=DCMbe,Vb
  Bus Selector3 : BusSelector  OutputSignals=Xe,Euler
  Constant4 : Constant  Value=0
  Constant5 : Constant  Value=0
  Gravity : Subsystem
  Propulsion : Subsystem
  Switch : Switch  Criteria=u2 > Threshold  SaturateOnIntegerOverflow=off  InputSameDT=off
  Switch1 : Switch  Criteria=u2 > Threshold  SaturateOnIntegerOverflow=off  InputSameDT=off
  Weather Model : Subsystem  Variant=on  VariantControl=Weather Model
  F : Outport
  M : Outport  Port=2
  RotorParams : Outport  Port=3
  AirData : Outport  Port=4
  wires:
  Bus Selector/1 -> Gravity/1(DCM_be), Aerodynamic Drag/1(DCM_be)  "<DCMbe>"
  Propulsion/3(F) -> Add/1
  Gravity/1(F_g) -> Add/2  "Gravity Force"
  Aerodynamic Drag/1(F_d) -> Add/4  "Drag Force"
  Bus Selector/2 -> Aerodynamic Drag/2(Vb)  "<Vb>"
  Add/1 -> F/1
  States/1 -> Bus Selector3/1, Bus Selector/1, Aerodynamic Forces/4(UAVState), Propulsion/2(States)  "States"
  CtrlSurfaces/1 -> Aerodynamic Forces/3(CtrlSurfaces)
  Add1/1 -> M/1
  Propulsion/2(M) -> Add1/2
  [AeroForce] -> Add/3  "Aerodynamic Force"
  Aerodynamic Forces/2(F) -> Switch/1
  Switch/1 -> [AeroForce]
  Constant4/1 -> Switch/3
  AeroSwitch/1 -> Switch/2, Switch1/2
  Constant5/1 -> Switch1/3
  Switch1/1 -> Add1/1, [AeroMoment]
  Aerodynamic Forces/3(M) -> Switch1/1
  Actuator/1 -> Propulsion/1(Actuator)
  Propulsion/1(RotorParameters) -> RotorParams/1
  Aerodynamic Forces/1(AirData) -> AirData/1, Weather Model/1(AirData)  "Air Data"
  Bus Selector3/1 -> Weather Model/2(Xe)  "<Xe>"
  Bus Selector3/2 -> Weather Model/3(Euler)  "<Euler>"
  Weather Model/1(Wind_e) -> Aerodynamic Forces/1(Wind_e)
  Weather Model/2(Rho) -> Aerodynamic Forces/2(Rho)

== system eVTOL_System/Dynamics/Ground Truth Bus ==
  Ve : Inport
  Xe : Inport  Port=2
  Euler : Inport  Port=3
  DCMbe : Inport  Port=4
  Vb : Inport  Port=5
  pqr : Inport  Port=6
  Abb : Inport  Port=7
  Abe : Inport  Port=8
  RotorParams : Inport  Port=9
  AirData : Inport  Port=10
  Bus Creator : BusCreator  Inputs=13
  Bus Selector : BusSelector  OutputSignals=airspeed
  Direction Cosine Matrix to Quaternions : sharedtransform/Direction Cosine Matrix  to Quaternions  aMode=0  action=None  tolerance=eps(2)
      settings: LibrarySourceBlock=|
      | aerolibtransform2/Direction Cosine Matrix
      | to Quaternions
  MATLAB Function1 : MATLAB Function  TreatAsAtomicUnit=on
  Ground Truth : Outport
  wires:
  pqr/1 -> Bus Creator/6
  Xe/1 -> Bus Creator/2
  Bus Creator/1 -> Ground Truth/1
  DCMbe/1 -> Direction Cosine Matrix to Quaternions/1, Bus Creator/4
  Euler/1 -> Bus Creator/3
  Vb/1 -> Bus Creator/5
  Abb/1 -> Bus Creator/7
  AirData/1 -> Bus Selector/1
  Bus Selector/1 -> Bus Creator/9  "<airspeed>"
  Direction Cosine Matrix to Quaternions/1 -> Bus Creator/10  "q"
  RotorParams/1 -> Bus Creator/8  "RotorParameters"
  Abe/1 -> Bus Creator/11  "Abe"
  MATLAB Function1/2(gndSpeed) -> Bus Creator/13  "gndspeed"
  MATLAB Function1/1(course) -> Bus Creator/12  "course"
  Ve/1 -> MATLAB Function1/1(vxyz), Bus Creator/1

== system eVTOL_System/Dynamics/Variant Subsystem ==
  UAVStates : Inport
  No Sensors : Subsystem  VariantControl=SensorType==0
  Sensors : Subsystem  VariantControl=SensorType==1
  SensorData : Outport

== system eVTOL_System/Flight Controller/Autopilot ==
  note: To modify the output bus interfaces, run open("exampleHelperDefineDigitalTwinInterface.m")
  HoverCommands : Inport
  FixedWingSP : Inport  Port=2
  AAC : Inport  Port=3
  CtrlMode : Inport  Port=4
  FlightMode : Inport  Port=5
  EstimatedStates : Inport  Port=6
  Bus Selector : BusSelector  OutputSignals=inTransition
  Bus Selector1 : BusSelector  OutputSignals=TransitionCondition
  Bus Selector2 : BusSelector  OutputSignals=w1,w2,w3,w4
  Filter or Estimator : Subsystem
  Fixed Wing Controller : Subsystem  Variant=on  VariantControl=Fixed Wing Controller
  Manual Control : Subsystem
  Multicopter Controller : Subsystem
  Scheduler : Subsystem  SystemSampleTime=0.005
  Scope : Scope  NumInputPorts=4
  Tilt Scheduler : Subsystem
  MotorActuatorCommands : Outport
  CtrlSurfaceCmds : Outport  Port=2
  wires:
  EstimatedStates/1 -> Filter or Estimator/1(SensorData)
  Multicopter Controller/1(MixerCommands) -> Scheduler/1(MotorCommands)
  Tilt Scheduler/1(TiltAngle) -> Scheduler/2(TiltSchedule)
  Fixed Wing Controller/1(Actuator) -> Scheduler/6(FixedWingActuators)
  CtrlMode/1 -> Bus Selector1/1, Fixed Wing Controller/2(Control Mode), Bus Selector/1
  Manual Control/1(AERT) -> Fixed Wing Controller/5(AERT)
  Scheduler/1(MotorActuatorCommands) -> Bus Selector2/1, MotorActuatorCommands/1
  Scheduler/2(CtrlSurfaceCommands) -> CtrlSurfaceCmds/1
  HoverCommands/1 -> Multicopter Controller/1(Hover Commands)
  FlightMode/1 -> Tilt Scheduler/1(FlightMode)
  Filter or Estimator/1(States) -> Multicopter Controller/3(States), Fixed Wing Controller/1(States), Tilt Scheduler/2(States), Scheduler/4(States)
  AAC/1 -> Fixed Wing Controller/3(AAC SP)
  FixedWingSP/1 -> Fixed Wing Controller/4(FixedWingSP)
  [TransitionDone] -> Scheduler/5(TransitionDone)
  Tilt Scheduler/2(FlightState) -> Scheduler/3(FlightState)
  Bus Selector/1 -> Multicopter Controller/2(InTransition)  "<inTransition>"
  Bus Selector1/1 -> [TransitionDone]  "<TransitionCondition>"
  Bus Selector2/1 -> Scope/1  "<w1>"
  Bus Selector2/2 -> Scope/2  "<w2>"
  Bus Selector2/3 -> Scope/3  "<w3>"
  Bus Selector2/4 -> Scope/4  "<w4>"

== system eVTOL_System/Flight Controller/Estimator ==
  SensorData : Inport
  Estimation Filter : Subsystem  VariantControl=SensorType==1
  Ground Truth : Subsystem  VariantControl=SensorType==0
  EstimatedStates : Outport

== system eVTOL_System/Flight Controller/Ground Control Station ==
  note: Set mission type. In the project shortcut, choose between:
      | Hover mission by selecting Guidance Mode under Hover
      | Fixed wing mission by selecting Guidance Mode under Fixed wing
      | Transition mission by selecting Set Up Full Transition Mission under Transition
      | City mission by selecting Set Up City Mission under Photorealistic Simulation
  UAVState : Inport
  Get Flight Mission : Subsystem  Variant=on  VariantControlMode=label  LabelModeActiveChoice=useQGC==0
  Global Mission : Outport
  wires:
  Get Flight Mission/1("Mission ") -> Global Mission/1
  UAVState/1 -> Get Flight Mission/1(UAVState)

== system eVTOL_System/Flight Controller/Guidance Test Bench ==
  note: Set control type. In the project shortcut, choose between:
      | 1. Manual control by selecting Manual Mode under Hover and open the subsystem to manually control the UAV in hover mode.
      | 2. Guidance testbench with prebuilt mission by selecting Guidance Mod e in the project shortcut.
  Aircraft States : Inport
  Global Mission : Inport  Port=2
  ControlType : Subsystem  Variant=on  VariantControl=Choice
  Rate Transition : RateTransition  OutPortSampleTime=0.005
  "Reference Tracking " : Subsystem
      settings: PortSchema="{\"entries\":[{\"content\":{\"sides\":[{\"content\":{\"connectorIds\":[\"In1\"]},\"type\":\"ConnectorPlacement.EquallySpacedRectSide\",\"uuid\":\"259d5f1e-a362-4dc0-8429-ef92dd781b31\"},{\"content\":{\"connectorIds\":[\"In2\",\"In3\"],\"side\":\"RIGHT\"},\"type\":\"ConnectorPlacement.EquallySpacedRectSide\",\"uuid\":\"8f699bfb-ab92-4bfa-94de-3c6c350a8a94\"},{\"content\":{\"connectorIds\":[],\"side\":\"TOP\"},\"type\":\"ConnectorPlacement.EquallySpacedRectSide\",\"uuid\":\"95dbffc6-e5b7-446a-adcb-afa0cff8c552\"}]},\"type\":\"ConnectorPlacement.EquallySpacedConnector\",\"uuid\":\"e657b5d9-4fa5-41f8-85e3-18a1074ff1cd\"}],\"packageUris\":[\"http://schema.mathworks.com/mf0/Connector/R2020b\"],\"version\":\"1.0\"}"
  HoverSP : Outport
  FixedWingSP : Outport  Port=2
  AACSP : Outport  Port=3
  ctrlMode : Outport  Port=4
  FlightMode : Outport  Port=5
  wires:
  Aircraft States/1 -> Rate Transition/1
  ControlType/1(HoverCmds) -> "Reference Tracking "/2(Position Command), HoverSP/1
  Global Mission/1 -> ControlType/2(Global Mission)
  ControlType/2(FixedWingSP) -> FixedWingSP/1
  ControlType/5(FlightMode) -> FlightMode/1
  ControlType/4(ctrlMode) -> ctrlMode/1
  ControlType/3(AACSP) -> "Reference Tracking "/3(AAC Commands), AACSP/1
  Rate Transition/1 -> "Reference Tracking "/1(State), ControlType/1(Aircraft States)

== system eVTOL_System/Motor Drive/Actuator To PWM for all motors ==
  Motor Commands : Inport
  Bus Creator : BusCreator  Inputs=6  OutDataTypeStr=Bus: RotorCntrlBus
  Bus Selector : BusSelector  OutputSignals=w1,w2,w3,w4,Tilt1,Tilt2
  Gain{,1..2,4} (4 alike) : Gain  Gain=1/(uavParam.motor.RPMMAX/60)
  Gain3 : Gain  Gain=1/(pi/2)
  Gain5 : Gain  Gain=1/(pi/2)
  To PWM : Outport
  wires:
  Motor Commands/1 -> Bus Selector/1
  Bus Selector/1 -> Gain/1  "<w1>"
  Bus Selector/3 -> Gain1/1  "<w3>"
  Bus Selector/2 -> Gain4/1  "<w2>"
  Bus Selector/4 -> Gain2/1  "<w4>"
  Bus Selector/5 -> Gain3/1  "<Tilt1>"
  Bus Selector/6 -> Gain5/1  "<Tilt2>"
  Gain/1 -> Bus Creator/1  "w1"
  Gain4/1 -> Bus Creator/2  "w2"
  Gain1/1 -> Bus Creator/3  "w3"
  Gain2/1 -> Bus Creator/4  "w4"
  Gain3/1 -> Bus Creator/5  "Tilt1"
  Gain5/1 -> Bus Creator/6  "Tilt2"
  Bus Creator/1 -> To PWM/1

== system eVTOL_System/Motor Drive/Actuator To RPM for 1 motor ==
  Motor Commands : Inport
  Gain : Gain  Gain=10
  Selector : Selector  InputPortWidth=6  IndexOptions=Index vector (dialog)  Indices=[1]  OutputSizes=1
  RPM : Outport
  wires:
  Motor Commands/1 -> Selector/1
  Selector/1 -> Gain/1
  Gain/1 -> RPM/1

== system eVTOL_System/Motor Drive/Actuator To RPM for 1 motor1 ==
  Motor Commands : Inport
  Gain : Gain  Gain=10
  Selector : Selector  InputPortWidth=6  IndexOptions=Index vector (dialog)  Indices=[2]  OutputSizes=1
  RPM : Outport
  wires:
  Motor Commands/1 -> Selector/1
  Selector/1 -> Gain/1
  Gain/1 -> RPM/1

== system eVTOL_System/Motor Drive/Actuator To RPM for 1 motor2 ==
  Motor Commands : Inport
  Gain : Gain  Gain=10
  Selector : Selector  InputPortWidth=6  IndexOptions=Index vector (dialog)  Indices=[3]  OutputSizes=1
  RPM : Outport
  wires:
  Motor Commands/1 -> Selector/1
  Selector/1 -> Gain/1
  Gain/1 -> RPM/1

== system eVTOL_System/Motor Drive/Actuator To RPM for 1 motor3 ==
  Motor Commands : Inport
  Gain : Gain  Gain=10
  Selector : Selector  InputPortWidth=6  IndexOptions=Index vector (dialog)  Indices=[4]  OutputSizes=1
  RPM : Outport
  wires:
  Motor Commands/1 -> Selector/1
  Selector/1 -> Gain/1
  Gain/1 -> RPM/1

== system eVTOL_System/Motor Drive/Controller ==
  Iab : Inport
  QAE_MIL_fbk : Inport  Port=2
  EnablePWM : Inport  Port=3
  Closed_Loop_FOC : Inport  Port=4
  Speed_CMD_RPM : Inport  Port=5
  Controller_Parameters : Inport  Port=6
  Controller_HIL_CAN : Subsystem  VariantControl=strcmp(get_param(['eVTOL_System/Motor Drive/SimulationVariant'], 'Value'),'3')
  Controller_MIL : Subsystem  VariantControl=(default)
  Controller_fbk : Outport
  Simu_config : Outport  Port=2

== system eVTOL_System/Motor Drive/Controller Parameters ==
  Controller_Parameters : BusCreator  Inputs=6
  Controller_Parameters1 : BusCreator  Inputs=6
  Default Values : Constant  OutDataTypeStr=boolean  SampleTime=Ts_UI
  Foc_Ki_S : Constant  Value=Foc_Ki_S  OutDataTypeStr=single
  Foc_Kp_I : Constant  Value=Foc_Kp_I  OutDataTypeStr=single
  Foc_Kp_S : Constant  Value=Foc_Kp_S  OutDataTypeStr=single
  Ia Offset : Constant  Value=Ia_offset  OutDataTypeStr=single
  Ia_offset : Constant  Value=Ia_offset  OutDataTypeStr=single  SampleTime=Ts_UI
  Ib Offset : Constant  Value=Ib_offset  OutDataTypeStr=single
  Ib_offset : Constant  Value=Ib_offset  OutDataTypeStr=single  SampleTime=Ts_UI
  Ki_S : Constant  Value=0.1  OutDataTypeStr=single  SampleTime=Ts_UI
  Ki_i*Tcpu : Constant  Value=Foc_Ki_IxTcpu  OutDataTypeStr=single  SampleTime=Ts_UI
  Ki_i*Tcpu1 : Constant  Value=Foc_Ki_IxTcpu  OutDataTypeStr=single
  Kp_I : Constant  Value=Foc_Kp_I  OutDataTypeStr=single  SampleTime=Ts_UI
  Kp_S : Constant  Value=0.1  OutDataTypeStr=single  SampleTime=Ts_UI
  Rate Transition : RateTransition  OutPortSampleTime=Ts_UI
  Switch : Switch  Criteria=u2 ~= 0  SaturateOnIntegerOverflow=off  InputSameDT=off
  Controller Parameters : Outport
  wires:
  Ia_offset/1 -> Controller_Parameters/5  "Ia_offset"
  Foc_Kp_S/1 -> Controller_Parameters1/1  "Kp_S"
  Ia Offset/1 -> Controller_Parameters1/5  "Ia_offset"
  Ib Offset/1 -> Controller_Parameters1/6  "Ib_offset"
  Controller_Parameters/1 -> Switch/3
  Foc_Ki_S/1 -> Controller_Parameters1/2  "Ki_S"
  Foc_Kp_I/1 -> Controller_Parameters1/3  "Kp_I"
  Controller_Parameters1/1 -> Rate Transition/1
  Ib_offset/1 -> Controller_Parameters/6  "Ib_offset"
  Ki_i*Tcpu/1 -> Controller_Parameters/4  "Ki_IxTcpu"
  Ki_S/1 -> Controller_Parameters/2  "Ki_S"
  Ki_i*Tcpu1/1 -> Controller_Parameters1/4  "Ki_IxTcpu"
  Kp_I/1 -> Controller_Parameters/3  "Kp_I"
  Kp_S/1 -> Controller_Parameters/1  "Kp_S"
  Switch/1 -> Controller Parameters/1
  Rate Transition/1 -> Switch/1
  Default Values/1 -> Switch/2  "Default Values"

== system eVTOL_System/Motor Drive/Controller Parameters1 ==
  Controller_Parameters : BusCreator  Inputs=6
  Controller_Parameters1 : BusCreator  Inputs=6
  Default Values : Constant  OutDataTypeStr=boolean  SampleTime=Ts_UI
  Foc_Ki_S : Constant  Value=Foc_Ki_S  OutDataTypeStr=single
  Foc_Kp_I : Constant  Value=Foc_Kp_I  OutDataTypeStr=single
  Foc_Kp_S : Constant  Value=Foc_Kp_S  OutDataTypeStr=single
  Ia Offset : Constant  Value=Ia_offset  OutDataTypeStr=single
  Ia_offset : Constant  Value=Ia_offset  OutDataTypeStr=single  SampleTime=Ts_UI
  Ib Offset : Constant  Value=Ib_offset  OutDataTypeStr=single
  Ib_offset : Constant  Value=Ib_offset  OutDataTypeStr=single  SampleTime=Ts_UI
  Ki_S : Constant  Value=0.1  OutDataTypeStr=single  SampleTime=Ts_UI
  Ki_i*Tcpu : Constant  Value=Foc_Ki_IxTcpu  OutDataTypeStr=single  SampleTime=Ts_UI
  Ki_i*Tcpu1 : Constant  Value=Foc_Ki_IxTcpu  OutDataTypeStr=single
  Kp_I : Constant  Value=Foc_Kp_I  OutDataTypeStr=single  SampleTime=Ts_UI
  Kp_S : Constant  Value=0.1  OutDataTypeStr=single  SampleTime=Ts_UI
  Rate Transition : RateTransition  OutPortSampleTime=Ts_UI
  Switch : Switch  Criteria=u2 ~= 0  SaturateOnIntegerOverflow=off  InputSameDT=off
  Controller Parameters : Outport
  wires:
  Ia_offset/1 -> Controller_Parameters/5  "Ia_offset"
  Foc_Kp_S/1 -> Controller_Parameters1/1  "Kp_S"
  Ia Offset/1 -> Controller_Parameters1/5  "Ia_offset"
  Ib Offset/1 -> Controller_Parameters1/6  "Ib_offset"
  Controller_Parameters/1 -> Switch/3
  Foc_Ki_S/1 -> Controller_Parameters1/2  "Ki_S"
  Foc_Kp_I/1 -> Controller_Parameters1/3  "Kp_I"
  Controller_Parameters1/1 -> Rate Transition/1
  Ib_offset/1 -> Controller_Parameters/6  "Ib_offset"
  Ki_i*Tcpu/1 -> Controller_Parameters/4  "Ki_IxTcpu"
  Ki_S/1 -> Controller_Parameters/2  "Ki_S"
  Ki_i*Tcpu1/1 -> Controller_Parameters1/4  "Ki_IxTcpu"
  Kp_I/1 -> Controller_Parameters/3  "Kp_I"
  Kp_S/1 -> Controller_Parameters/1  "Kp_S"
  Switch/1 -> Controller Parameters/1
  Rate Transition/1 -> Switch/1
  Default Values/1 -> Switch/2  "Default Values"

== system eVTOL_System/Motor Drive/Controller Parameters2 ==
  Controller_Parameters : BusCreator  Inputs=6
  Controller_Parameters1 : BusCreator  Inputs=6
  Default Values : Constant  OutDataTypeStr=boolean  SampleTime=Ts_UI
  Foc_Ki_S : Constant  Value=Foc_Ki_S  OutDataTypeStr=single
  Foc_Kp_I : Constant  Value=Foc_Kp_I  OutDataTypeStr=single
  Foc_Kp_S : Constant  Value=Foc_Kp_S  OutDataTypeStr=single
  Ia Offset : Constant  Value=Ia_offset  OutDataTypeStr=single
  Ia_offset : Constant  Value=Ia_offset  OutDataTypeStr=single  SampleTime=Ts_UI
  Ib Offset : Constant  Value=Ib_offset  OutDataTypeStr=single
  Ib_offset : Constant  Value=Ib_offset  OutDataTypeStr=single  SampleTime=Ts_UI
  Ki_S : Constant  Value=0.1  OutDataTypeStr=single  SampleTime=Ts_UI
  Ki_i*Tcpu : Constant  Value=Foc_Ki_IxTcpu  OutDataTypeStr=single  SampleTime=Ts_UI
  Ki_i*Tcpu1 : Constant  Value=Foc_Ki_IxTcpu  OutDataTypeStr=single
  Kp_I : Constant  Value=Foc_Kp_I  OutDataTypeStr=single  SampleTime=Ts_UI
  Kp_S : Constant  Value=0.1  OutDataTypeStr=single  SampleTime=Ts_UI
  Rate Transition : RateTransition  OutPortSampleTime=Ts_UI
  Switch : Switch  Criteria=u2 ~= 0  SaturateOnIntegerOverflow=off  InputSameDT=off
  Controller Parameters : Outport
  wires:
  Ia_offset/1 -> Controller_Parameters/5  "Ia_offset"
  Foc_Kp_S/1 -> Controller_Parameters1/1  "Kp_S"
  Ia Offset/1 -> Controller_Parameters1/5  "Ia_offset"
  Ib Offset/1 -> Controller_Parameters1/6  "Ib_offset"
  Controller_Parameters/1 -> Switch/3
  Foc_Ki_S/1 -> Controller_Parameters1/2  "Ki_S"
  Foc_Kp_I/1 -> Controller_Parameters1/3  "Kp_I"
  Controller_Parameters1/1 -> Rate Transition/1
  Ib_offset/1 -> Controller_Parameters/6  "Ib_offset"
  Ki_i*Tcpu/1 -> Controller_Parameters/4  "Ki_IxTcpu"
  Ki_S/1 -> Controller_Parameters/2  "Ki_S"
  Ki_i*Tcpu1/1 -> Controller_Parameters1/4  "Ki_IxTcpu"
  Kp_I/1 -> Controller_Parameters/3  "Kp_I"
  Kp_S/1 -> Controller_Parameters/1  "Kp_S"
  Switch/1 -> Controller Parameters/1
  Rate Transition/1 -> Switch/1
  Default Values/1 -> Switch/2  "Default Values"

== system eVTOL_System/Motor Drive/Controller Parameters3 ==
  Controller_Parameters : BusCreator  Inputs=6
  Controller_Parameters1 : BusCreator  Inputs=6
  Default Values : Constant  OutDataTypeStr=boolean  SampleTime=Ts_UI
  Foc_Ki_S : Constant  Value=Foc_Ki_S  OutDataTypeStr=single
  Foc_Kp_I : Constant  Value=Foc_Kp_I  OutDataTypeStr=single
  Foc_Kp_S : Constant  Value=Foc_Kp_S  OutDataTypeStr=single
  Ia Offset : Constant  Value=Ia_offset  OutDataTypeStr=single
  Ia_offset : Constant  Value=Ia_offset  OutDataTypeStr=single  SampleTime=Ts_UI
  Ib Offset : Constant  Value=Ib_offset  OutDataTypeStr=single
  Ib_offset : Constant  Value=Ib_offset  OutDataTypeStr=single  SampleTime=Ts_UI
  Ki_S : Constant  Value=0.1  OutDataTypeStr=single  SampleTime=Ts_UI
  Ki_i*Tcpu : Constant  Value=Foc_Ki_IxTcpu  OutDataTypeStr=single  SampleTime=Ts_UI
  Ki_i*Tcpu1 : Constant  Value=Foc_Ki_IxTcpu  OutDataTypeStr=single
  Kp_I : Constant  Value=Foc_Kp_I  OutDataTypeStr=single  SampleTime=Ts_UI
  Kp_S : Constant  Value=0.1  OutDataTypeStr=single  SampleTime=Ts_UI
  Rate Transition : RateTransition  OutPortSampleTime=Ts_UI
  Switch : Switch  Criteria=u2 ~= 0  SaturateOnIntegerOverflow=off  InputSameDT=off
  Controller Parameters : Outport
  wires:
  Ia_offset/1 -> Controller_Parameters/5  "Ia_offset"
  Foc_Kp_S/1 -> Controller_Parameters1/1  "Kp_S"
  Ia Offset/1 -> Controller_Parameters1/5  "Ia_offset"
  Ib Offset/1 -> Controller_Parameters1/6  "Ib_offset"
  Controller_Parameters/1 -> Switch/3
  Foc_Ki_S/1 -> Controller_Parameters1/2  "Ki_S"
  Foc_Kp_I/1 -> Controller_Parameters1/3  "Kp_I"
  Controller_Parameters1/1 -> Rate Transition/1
  Ib_offset/1 -> Controller_Parameters/6  "Ib_offset"
  Ki_i*Tcpu/1 -> Controller_Parameters/4  "Ki_IxTcpu"
  Ki_S/1 -> Controller_Parameters/2  "Ki_S"
  Ki_i*Tcpu1/1 -> Controller_Parameters1/4  "Ki_IxTcpu"
  Kp_I/1 -> Controller_Parameters/3  "Kp_I"
  Kp_S/1 -> Controller_Parameters/1  "Kp_S"
  Switch/1 -> Controller Parameters/1
  Rate Transition/1 -> Switch/1
  Default Values/1 -> Switch/2  "Default Values"

== system eVTOL_System/Motor Drive/Controller1 ==
  Iab : Inport
  QAE_MIL_fbk : Inport  Port=2
  EnablePWM : Inport  Port=3
  Closed_Loop_FOC : Inport  Port=4
  Speed_CMD_RPM : Inport  Port=5
  Controller_Parameters : Inport  Port=6
  Controller_MIL : Subsystem  VariantControl=(default)
  Controller_fbk : Outport
  Simu_config : Outport  Port=2

== system eVTOL_System/Motor Drive/Controller2 ==
  Iab : Inport
  QAE_MIL_fbk : Inport  Port=2
  EnablePWM : Inport  Port=3
  Closed_Loop_FOC : Inport  Port=4
  Speed_CMD_RPM : Inport  Port=5
  Controller_Parameters : Inport  Port=6
  Controller_MIL : Subsystem  VariantControl=(default)
  Controller_fbk : Outport
  Simu_config : Outport  Port=2
